simulink model "First_order_integrator_method"  (R2024a)
settings: Solver=VariableStepAuto  StartTime=0.0  StopTime=10.0  RelTol=1e-3
values from neighbouring files (symbols this model uses):
  b = 100    [First_order_parameters.mat]
  j = 10    [First_order_parameters.mat]
  k = 5000    [First_order_parameters.mat]
settings Model: Creator=nassa  LastModifiedBy=nassa

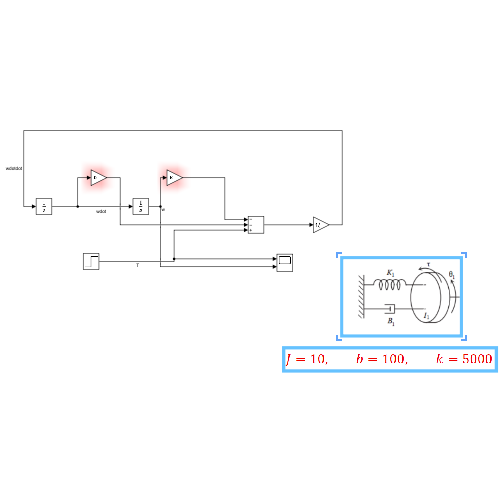
[thumbnail: Simulink's stored preview of the top-level diagram]
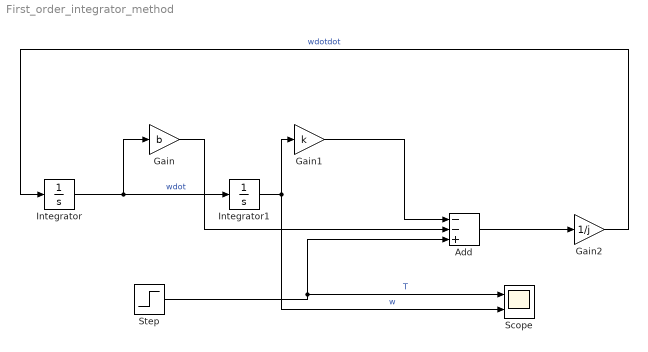
== system First_order_integrator_method ==
  Add : Sum  Inputs=--+
  Gain : Gain  Gain=b
  Gain1 : Gain  Gain=k
  Gain2 : Gain  Gain=1/j
  Integrator : Integrator
  Integrator1 : Integrator
  Scope : Scope  NumInputPorts=2
  Step : Step  SampleTime=0
  wires:
  Integrator/1 -> Gain/1, Integrator1/1  "wdot"
  Integrator1/1 -> Scope/2, Gain1/1  "w"
  Gain2/1 -> Integrator/1  "wdotdot"
  Gain1/1 -> Add/1
  Gain/1 -> Add/2
  Step/1 -> Scope/1, Add/3  "T"
  Add/1 -> Gain2/1
